simulink model "LandingGear"  (R2017b)
settings: Solver=VariableStepAuto  StartTime=0.0  StopTime=10.0  RelTol=1e-3
settings Model: Creator=zht  LastModifiedBy=zht

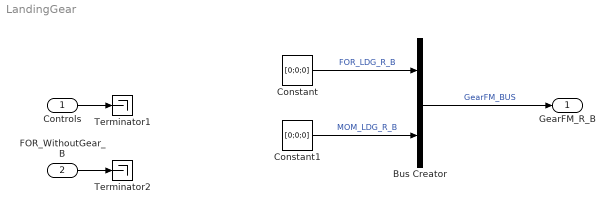
== system LandingGear ==
  Controls : Inport  OutDataTypeStr=Bus: RC_In_BUS
  FOR_WithoutGear_B : Inport  Port=2
  Bus Creator : BusCreator  Inputs=2  OutDataTypeStr=Bus: GearFM_BUS
  Constant : Constant  Value=[0;0;0]
  Constant1 : Constant  Value=[0;0;0]
  Terminator1 : Terminator
  Terminator2 : Terminator
  GearFM_R_B : Outport  OutDataTypeStr=Bus: GearFM_BUS
  wires:
  Bus Creator/1 -> GearFM_R_B/1  "GearFM_BUS"
  Constant1/1 -> Bus Creator/2  "MOM_LDG_R_B"
  Constant/1 -> Bus Creator/1  "FOR_LDG_R_B"
  Controls/1 -> Terminator1/1
  FOR_WithoutGear_B/1 -> Terminator2/1
